simulink model "SUPER_CAPACITOR"  (R2016a)
settings: Solver=VariableStepAuto  StartTime=0.0  StopTime=0.3  MaxStep=1e-7  RelTol=1e-3
InitFcn:
  | Ts=1e-6
libraries: powerlib x24, simulink x3, powerlib_meascontrol x3, electricdrivelib x1, powerlib_extras x1
settings Model: Creator=KARTHIK  LastModifiedBy=kalla
settings SolverCC: ZeroCrossControl=DisableAll

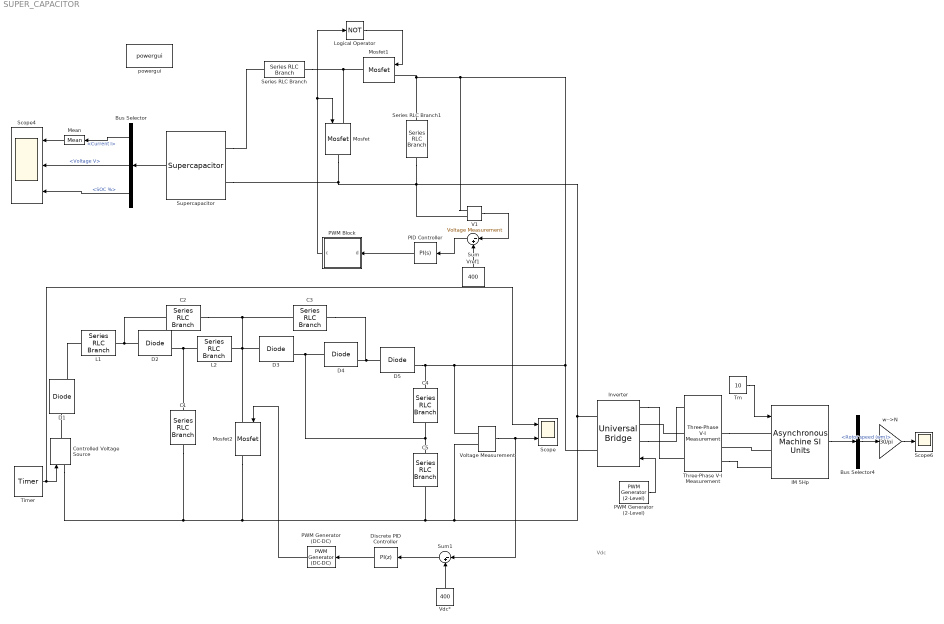
== system SUPER_CAPACITOR ==
  note: Vdc
  Bus Selector : BusSelector  OutputSignals=Current I,Voltage V,SOC %
  Bus Selector4 : BusSelector  OutputSignals=Mechanical.Rotor speed (wm)
  C{1,3..5} (4 alike) : powerlib/Elements/Series RLC Branch  LConnTagsString=__new0  RConnTagsString=__new0  BranchType=C  Resistance=1  Inductance=1e-3  SetiL0=off  InitialCurrent=0  Capacitance=520e-6  Setx0=off  InitialVoltage=0  Measurements=Branch voltage
  C2 : powerlib/Elements/Series RLC Branch  LConnTagsString=__new0  RConnTagsString=__new0  BranchType=C  Resistance=1  Inductance=1e-3  SetiL0=off  InitialCurrent=0  Capacitance=780e-6  Setx0=off  InitialVoltage=0  Measurements=Branch voltage
  Controlled Voltage Source : powerlib/Electrical Sources/Controlled Voltage Source  Initialize=on  Source_Type=AC  Amplitude=0  Phase=0  Frequency=0  Measurements=None
  D{1..5} (5 alike) : powerlib/Power Electronics/Diode  Ron=0.001  Lon=0  Vf=0.8  IC=0  UseSnubber=off  Rs=500  Cs=250e-9  Measurements=on
  Discrete PID Controller : simulink/Continuous/PID Controller  Controller=PI  TimeDomain=Discrete-time  SampleTime=1e-5  IntegratorMethod=Forward Euler  FilterMethod=Forward Euler  Form=Parallel  UseFilter=on  ControllerParametersSource=internal  P=0.0001  I=0.0005  D=0  N=100  InitialConditionSource=internal  InitialConditionForIntegrator=0  InitialConditionForFilter=0  ExternalReset=none  LimitOutput=on  UpperSaturationLimit=0.5  LowerSaturationLimit=0  LinearizeAsGain=off  AntiWindupMode=none  Kb=1  TrackingMode=off  Kt=1  PParamMin=[]  PParamMax=[]  IParamMin=[]  IParamMax=[]  DParamMin=[]  DParamMax=[]  NParamMin=[]  NParamMax=[]  KbParamMin=[]  KbParamMax=[]  KtParamMin=[]  KtParamMax=[]  POutMin=[]  POutMax=[]  IOutMin=[]  IOutMax=[]  DOutMin=[]  DOutMax=[]  NOutMin=[]  NOutMax=[]  KbOutMin=[]  KbOutMax=[]  KtOutMin=[]  KtOutMax=[]  IntegratorOutMin=[]  IntegratorOutMax=[]  FilterOutMin=[]  FilterOutMax=[]  SumOutMin=[]  SumOutMax=[]  SumI1OutMin=[]  SumI1OutMax=[]  SumI2OutMin=[]  SumI2OutMax=[]  SumI3OutMin=[]  SumI3OutMax=[]  SumDOutMin=[]  SumDOutMax=[]  SaturationOutMin=[]  SaturationOutMax=[]  IntegratorContinuousStateAttributes=''  IntegratorStateMustResolveToSignalObject=off  IntegratorRTWStateStorageClass=Auto  FilterContinuousStateAttributes=''  FilterStateMustResolveToSignalObject=off  FilterRTWStateStorageClass=Auto  DifferentiatorICPrevScaledInput=0  DifferentiatorOutMin=[]  DifferentiatorOutMax=[]
  IM 5Hp : powerlib/Machines/Asynchronous Machine SI Units  RotorType=Squirrel-cage  PresetModel="15:  5.4 HP (4KW)   400 V  50Hz 1430 RPM"  MechanicalLoad=Torque Tm  ShowDetailedParameters=on  ReferenceFrame=Rotor  Units=SI  MeasurementBus=off  NominalParameters=[4000 400 50]  Stator=[1.405 0.005839]  Rotor=[1.395 0.005839]  Cage1=[0.4155 0.002066]  Cage2=[0.4168 0.0003495]  Lm=0.1722  Mechanical=[0.0131 0.002985 2]  PolePairs=2  InitialConditions=[0 0 0 0 0 0 0 0]  SimulateSaturation=off  Saturation=[14.03593122, 27.81365428, 53.79336849, 72.68890987, 97.98006896, 148.6815601, 215.7428561, 302.9841135, 428.7778367 ; 230, 322, 414, 460, 506, 552, 598, 644, 690]  LoadFlowParameters=1492000  TsPowergui=0  TsBlock=-1  IterativeModel=Trapezoidal non iterative  IterativeDiscreteModel=Trapezoidal non iterative  Pmec=1.492e+006
  Inverter : powerlib/Power Electronics/Universal Bridge  Arms=3  SnubberResistance=1e5  SnubberCapacitance=inf  Device=IGBT / Diodes  Ron=1e-3  Lon=0  ForwardVoltages="[  0  0  ]"  ForwardVoltage=0  GTOparameters=[ 10e-6 , 20e-6 ]  IGBTparameters=[ 1e-6 , 2e-6 ]  Measurements=None  Measurements_2=None  converterType=Rectifier
  L1 : powerlib/Elements/Series RLC Branch  LConnTagsString=__new0  RConnTagsString=__new0  BranchType=L  Resistance=1  Inductance=323e-6  SetiL0=off  InitialCurrent=0  Capacitance=1e-6  Setx0=off  InitialVoltage=0  Measurements=Branch current
  L2 : powerlib/Elements/Series RLC Branch  LConnTagsString=__new0  RConnTagsString=__new0  BranchType=L  Resistance=1  Inductance=318e-6  SetiL0=off  InitialCurrent=0  Capacitance=1e-6  Setx0=off  InitialVoltage=0  Measurements=Branch current
  Logical Operator : Logic  Operator=NOT  AllPortsSameDT=off  OutDataTypeStr=boolean
  Mean : powerlib_meascontrol/Measurements/Mean  Freq=50  Vinit=0  Ts=Ts
  Mosfet : powerlib/Power Electronics/Mosfet  Ron=0.1  Lon=0  Rd=0.01  Vfd=0  IC=0  Rs=1e5  Cs=inf  Measurements=off
  Mosfet1 : powerlib/Power Electronics/Mosfet  Ron=0.1  Lon=0  Rd=0.01  Vfd=0  IC=0  Rs=1e5  Cs=inf  Measurements=off
  Mosfet2 : powerlib/Power Electronics/Mosfet  Ron=0.1  Lon=0  Rd=0.01  Vfd=0  IC=0  Rs=1e5  Cs=inf  Measurements=on
  PID Controller : simulink/Continuous/PID Controller  Controller=PI  TimeDomain=Continuous-time  SampleTime=-1  IntegratorMethod=Forward Euler  FilterMethod=Forward Euler  Form=Parallel  UseFilter=on  ControllerParametersSource=internal  P=0.1  I=0.00023  D=0  N=100  InitialConditionSource=internal  InitialConditionForIntegrator=0  InitialConditionForFilter=0  ExternalReset=none  LimitOutput=on  UpperSaturationLimit=0.85  LowerSaturationLimit=0  LinearizeAsGain=on  AntiWindupMode=none  Kb=1  TrackingMode=off  Kt=1  PParamMin=[]  PParamMax=[]  IParamMin=[]  IParamMax=[]  DParamMin=[]  DParamMax=[]  NParamMin=[]  NParamMax=[]  KbParamMin=[]  KbParamMax=[]  KtParamMin=[]  KtParamMax=[]  POutMin=[]  POutMax=[]  IOutMin=[]  IOutMax=[]  DOutMin=[]  DOutMax=[]  NOutMin=[]  NOutMax=[]  KbOutMin=[]  KbOutMax=[]  KtOutMin=[]  KtOutMax=[]  IntegratorOutMin=[]  IntegratorOutMax=[]  FilterOutMin=[]  FilterOutMax=[]  SumOutMin=[]  SumOutMax=[]  SumI1OutMin=[]  SumI1OutMax=[]  SumI2OutMin=[]  SumI2OutMax=[]  SumI3OutMin=[]  SumI3OutMax=[]  SumDOutMin=[]  SumDOutMax=[]  SaturationOutMin=[]  SaturationOutMax=[]  IntegratorContinuousStateAttributes=''  IntegratorStateMustResolveToSignalObject=off  IntegratorRTWStateStorageClass=Auto  FilterContinuousStateAttributes=''  FilterStateMustResolveToSignalObject=off  FilterRTWStateStorageClass=Auto  DifferentiatorICPrevScaledInput=0  DifferentiatorOutMin=[]  DifferentiatorOutMax=[]
  PWM Block : Subsystem  mask{fs=100e3}
      mask prompts: fs "Switching fFrequency"
  PWM Generator (2-Level) : powerlib_meascontrol/Pulse & Signal Generators/PWM Generator (2-Level)  ModulatorType=Three-phase bridge (6 pulses)  ModulatorMode=Unsynchronized  Fc=5000  Pc=0  nF=27  MinMax="[ -1  1 ]"  SamplingTechnique=Natural  ModulatingSignals=on  m=0.89  Freq=50  Phase=0  Ts=1e-5  ShowCarrierOutport=off
  PWM Generator (DC-DC) : powerlib_meascontrol/Pulse & Signal Generators/PWM Generator (DC-DC)  Fsw=20e3  Ts=1e-5
  Scope : Scope  NumInputPorts=2
  Scope4 : Scope  NumInputPorts=3
  Scope6 : Scope
  Series RLC Branch : powerlib/Elements/Series RLC Branch  LConnTagsString=__new0  RConnTagsString=__new0  BranchType=RL  Resistance=80e-3  Inductance=161.95e-6  SetiL0=off  InitialCurrent=0  Capacitance=1e-6  Setx0=off  InitialVoltage=0  Measurements=None
  Series RLC Branch1 : powerlib/Elements/Series RLC Branch  LConnTagsString=__new0  RConnTagsString=__new0  BranchType=RC  Resistance=5e-3  Inductance=1e-3  SetiL0=off  InitialCurrent=0  Capacitance=220e-6  Setx0=off  InitialVoltage=0  Measurements=None
  Sum : Sum  Inputs=|-+
  Sum1 : Sum  Inputs=|-+
  Supercapacitor : electricdrivelib/Extra Sources/Supercapacitor  C=99.5  Rdc=8.9e-3  Voltage=250  Ns=1  Np=1  Vinit=240  Temp=25  PresetModel=off  EstParam=off  Nc=1  r=1e-9  epsilon=6.0208e-10  Ich=10  Vstern="[0.161  2.7  7.8]"  Self_dis=on  Ioc=10  Vself="[48  47.8  47.06  44.65]"  demandeplot=off  I="[10  20 100  500]"  Units=sec  Vmax=0  If=0  deltaV=0  alpha=0  sec=0
  Three-Phase V-I Measurement : powerlib/Measurements/Three-Phase V-I Measurement  VoltageMeasurement=phase-to-phase  SetLabelV=off  LabelV=Vabc  Vpu=off  VpuLL=off  CurrentMeasurement=yes  SetLabelI=off  LabelI=Iabc  Ipu=off  Pbase=100e6  Vbase=500e3  OutputType=Complex  PhasorSimulation=off  PSBequivalent=0
  Timer : powerlib_extras/Control  Blocks/Timer  t=[0 0.1 0.2 0.3]  e=[150 50 100 150]
  Tm : Constant  Value=10
  V1 : powerlib/Measurements/Voltage Measurement  PhasorSimulation=off  OutputType=Complex  PSBequivalent=0
  Vdc* : Constant  Value=400
  Voltage Measurement : powerlib/Measurements/Voltage Measurement  PhasorSimulation=off  OutputType=Complex  PSBequivalent=0
  Vref1 : Constant  Value=400
  powergui : powerlib/powergui  Priority=1  SimulationMode=Continuous  SolverType=Tustin  SampleTime=1e-8  frequency=60  SPID=off  DisableSnubberDevices=off  DisableRonSwitches=off  DisableVfSwitches=off  SwTol=0  DisplayEquations=off  Interpol=off  ExternalGateDelay=off  methode=off  Ts=0  FunctionMessages=off  echomessages=off  HookPort=off  EnableUseOfTLC=off  x0status=blocks  frequencyindice=0  Pbase=100e6  ErrMax=1e-4  Iterations=50  UnitsV=kV  UnitsW=MW  buscounter=0  RestoreLinks=warning  ResistiveCurrentMeasurement=off  Frange=[0:2:500]  Ylog=off  Xlog=on  ShowGrid=off  save=off  variable=ZData  structure=tpa14cfcc1_35b5_40eb_8b70_049b43167a68  ZoomFFT=off  StartTime=0.0  cycles=1  DisplayStyle=1  fundamental=60  FreqAxis=off  MaxFrequency=1000  frequencyindicesteady=1  RmsSteady=1  display=off
  w-->N : Gain  Gain=30/pi
  wires:
  Logical Operator/1 -> Mosfet1/1
  PWM Block/1(c) -> Logical Operator/1, Mosfet/1
  V1/1 -> Sum/1
  Vref1/1 -> Sum/2
  Sum/1 -> PID Controller/1
  PID Controller/1 -> PWM Block/1(d)
  Supercapacitor/1 -> Bus Selector/1
  Bus Selector/1 -> Mean/1  "<Current I>"
  Bus Selector/2 -> Scope4/2  "<Voltage V>"
  Bus Selector/3 -> Scope4/3  "<SOC %>"
  Voltage Measurement/1 -> Scope/2, Sum1/1
  Vdc*/1 -> Sum1/2
  Sum1/1 -> Discrete PID Controller/1
  Discrete PID Controller/1 -> PWM Generator (DC-DC)/1
  PWM Generator (DC-DC)/1 -> Mosfet2/1
  Timer/1 -> Controlled Voltage Source/1, Scope/1
  Tm/1 -> IM 5Hp/1
  PWM Generator (2-Level)/1 -> Inverter/1
  IM 5Hp/1 -> Bus Selector4/1
  Bus Selector4/1 -> w-->N/1  "<Rotor speed (wm)>"
  w-->N/1 -> Scope6/1
  Mean/1 -> Scope4/1
  connections:
  Mosfet1/RConn1 -- Series RLC Branch/RConn1 -- Mosfet/LConn1
  Supercapacitor/LConn1 -- Series RLC Branch/LConn1
  L1/RConn1 -- D2/LConn1 -- C2/RConn1
  D2/RConn1 -- L2/LConn1 -- C1/LConn1
  Mosfet2/LConn1 -- C3/RConn1 -- C2/LConn1 -- D3/LConn1 -- L2/RConn1
  D4/RConn1 -- D5/LConn1 -- C3/LConn1
  Series RLC Branch1/LConn1 -- Mosfet1/LConn1 -- V1/LConn1 -- Inverter/RConn1 -- Voltage Measurement/LConn1 -- D5/RConn1 -- C4/LConn1
  Series RLC Branch1/RConn1 -- Mosfet/RConn1 -- Supercapacitor/LConn2 -- Inverter/RConn2 -- Voltage Measurement/LConn2 -- Controlled Voltage Source/LConn1 -- C1/RConn1 -- Mosfet2/RConn1 -- C5/RConn1 -- V1/LConn2
  D3/RConn1 -- D4/LConn1 -- C5/LConn1 -- C4/RConn1
  Three-Phase V-I Measurement/RConn3 -- IM 5Hp/LConn3
  Inverter/LConn1 -- Three-Phase V-I Measurement/LConn1
  L1/LConn1 -- D1/RConn1
  Three-Phase V-I Measurement/RConn1 -- IM 5Hp/LConn1
  Inverter/LConn3 -- Three-Phase V-I Measurement/LConn3
  IM 5Hp/LConn2 -- Three-Phase V-I Measurement/RConn2
  Three-Phase V-I Measurement/LConn2 -- Inverter/LConn2
  Controlled Voltage Source/RConn1 -- D1/LConn1

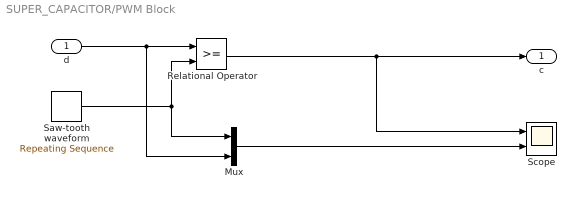
== system SUPER_CAPACITOR/PWM Block ==
  d : Inport
  Mux : Mux  Inputs=2
  Relational Operator : RelationalOperator  OutDataTypeStr=boolean
  Saw-tooth waveform : simulink/Sources/Repeating Sequence  rep_seq_t=[0 1/fs]  rep_seq_y=[0 1]
  Scope : Scope  NumInputPorts=2
  c : Outport
  wires:
  d/1 -> Mux/2, Relational Operator/1
  Saw-tooth waveform/1 -> Mux/1, Relational Operator/2
  Relational Operator/1 -> c/1, Scope/1
  Mux/1 -> Scope/2
